simulink subsystem "Nozzle"  (R2020b)
settings: Solver=VariableStepAuto  StartTime=0.0  StopTime=10.0  RelTol=1e-3
undefined symbols (not defined in the file or in its folder): Sim
settings Model: Creator=Edward  LastModifiedBy=Edward

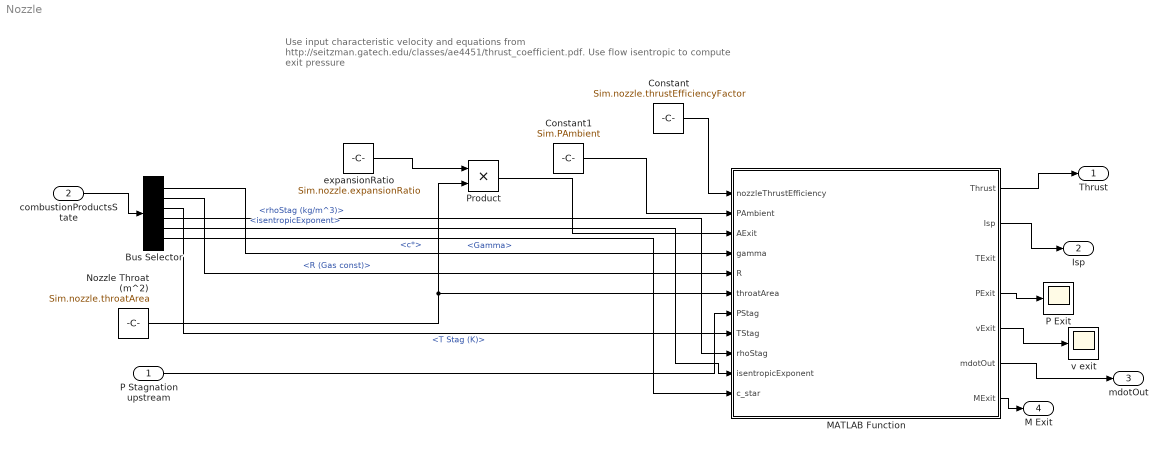
== system Nozzle ==
  note: Use input characteristic velocity and equations from http://seitzman.gatech.edu/classes/ae4451/thrust_coefficient.pdf.
      |
      | Use flow isentropic to compute exit pressure
  P Stagnation upstream : Inport
  combustionProductsState : Inport  Port=2
  Bus Selector : BusSelector  OutputSignals=Gamma,R (Gas const),T Stag (K),rhoStag (kg/m^3),isentropicExponent,c*
  Constant : Constant  Value=Sim.nozzle.thrustEfficiencyFactor
  Constant1 : Constant  Value=Sim.PAmbient
  MATLAB Function : MATLAB Function  TreatAsAtomicUnit=on
  Nozzle Throat (m^2) : Constant  Value=Sim.nozzle.throatArea
  "P Exit " : Scope
  Product : Product
  "expansionRatio " : Constant  Value=Sim.nozzle.expansionRatio
  v exit : Scope
  Thrust : Outport
  Isp : Outport  Port=2
  mdotOut : Outport  Port=3
  M Exit : Outport  Port=4
  wires:
  Bus Selector/3 -> MATLAB Function/8(TStag)  "<T Stag (K)>"
  Bus Selector/2 -> MATLAB Function/5(R)  "<R (Gas const)>"
  Bus Selector/1 -> MATLAB Function/4(gamma)  "<Gamma>"
  combustionProductsState/1 -> Bus Selector/1
  "expansionRatio "/1 -> Product/1
  Nozzle Throat (m^2)/1 -> MATLAB Function/6(throatArea), Product/2
  P Stagnation upstream/1 -> MATLAB Function/7(PStag)
  MATLAB Function/1(Thrust) -> Thrust/1
  MATLAB Function/2(Isp) -> Isp/1
  Constant/1 -> MATLAB Function/1(nozzleThrustEfficiency)
  Product/1 -> MATLAB Function/3(AExit)
  Constant1/1 -> MATLAB Function/2(PAmbient)
  MATLAB Function/6(mdotOut) -> mdotOut/1
  Bus Selector/4 -> MATLAB Function/9(rhoStag)  "<rhoStag (kg/m^3)>"
  MATLAB Function/4(PExit) -> "P Exit "/1
  MATLAB Function/5(vExit) -> v exit/1
  Bus Selector/6 -> MATLAB Function/11(c_star)  "<c*>"
  MATLAB Function/7(MExit) -> M Exit/1
  Bus Selector/5 -> MATLAB Function/10(isentropicExponent)  "<isentropicExponent>"

== matlab function Nozzle/MATLAB Function ==
  data: nozzleThrustEfficiency input; PAmbient input; AExit input; Thrust output; Isp output; TExit output; gamma input; R input; throatArea input; PStag input; TStag input; rhoStag input; isentropicExponent input; PExit output; vExit output; mdotOut output; c_star input; MExit output
function [Thrust, Isp, TExit, PExit, vExit, mdotOut, MExit] = thrustFunction(nozzleThrustEfficiency, ...
    PAmbient, AExit, gamma, R, throatArea, PStag, TStag, ...
    rhoStag, isentropicExponent, c_star)
coder.extrinsic('flowisentropic'); %flowisentropic doesn't support codegen
%Initialize variables so types are determined
MExit = 0;
TRatio = 0;
PRatio = 0;
rhoRatio = 0;
[MExit, TRatio, PRatio, rhoRatioIsentropic, ~] = flowisentropic(isentropicExponent, AExit./throatArea, 'sup');

TExit = TStag .* TRatio;
PExit = PStag .* PRatio;
vExit = MExit .* sqrt(gamma .* R .* TExit); %Isentropic so not quite in agreement with thrust calculation which has correction terms applied


%Using equations from:
%Rocket propulsion elements (Section on nozzles)
%http://seitzman.gatech.edu/classes/ae4451/thrust_coefficient.pdf
thrustCoeff = nozzleThrustEfficiency.*gamma.*sqrt( ...
    ((2./(gamma-1)) .* (2./(gamma+1)).^( (gamma+1)./(gamma-1) )) ...
    .*(1-(PExit./PStag).^( (gamma-1)./gamma )) ...
        ) ...
    + (PExit./PStag - PAmbient./PStag).*(AExit./throatArea);
mdotOut = (PStag.*throatArea)./c_star;
vExitEffective = thrustCoeff.*c_star;
Thrust = mdotOut.*vExitEffective;
Isp = Thrust ./ (mdotOut .* 9.81);
